simulink model "Remus_AUV_twin"  (R2025b)
settings: Solver=ode4  StartTime=0  StopTime=300  FixedStep=0.1  RelTol=1e-3
undefined symbols (not defined in the file): DiscIntNeverNeededParam
libraries: simulink x1, rllib x1
settings Model: Creator=usdas  LastModifiedBy=OMEN
settings DataIOCC: SaveState=on  InspectSignalLogs=on  ReturnWorkspaceOutputs=off  OutputSaveName=out

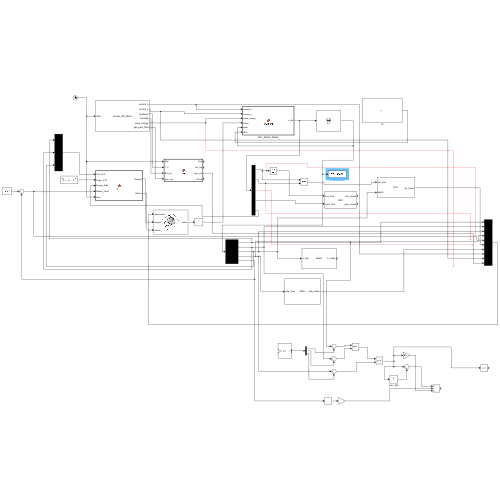
[thumbnail: Simulink's stored preview of the top-level diagram]
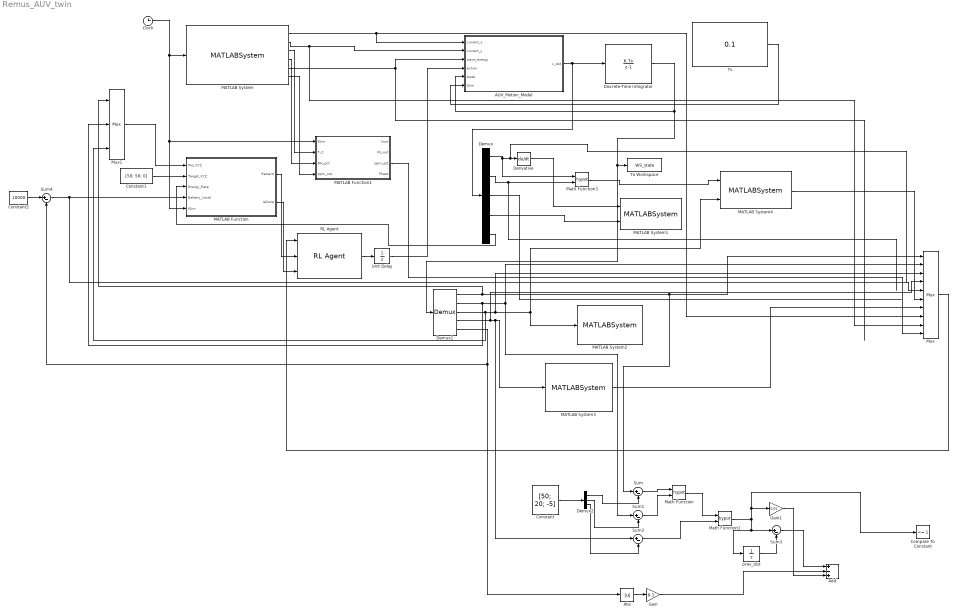
== system Remus_AUV_twin ==
  AUV_Motion_Model : MATLAB Function  TreatAsAtomicUnit=on
  Abs : Abs  SaturateOnIntegerOverflow=off
  Add : Sum  Inputs=+-+
  Clock : Clock
  Compare To Constant : simulink/Logic and Bit Operations/Compare To Constant  relop=<=  const=1  OutDataTypeStr=boolean
  Constant : Constant  Value=[50; 20; -5]  OutDataTypeStr=double  SampleTime=-1
  Constant1 : Constant  Value=[50; 50; 0]
  Constant2 : Constant  Value=10000
  Demux : Demux  Outputs=5
  Demux1 : Demux  Outputs=5
  Demux2 : Demux  Outputs=3
  Derivative : Derivative
  Discrete-Time Integrator : DiscreteIntegrator  InitialCondition=[1;1;0;0;0]  SampleTime=0.1  ICPrevOutput=DiscIntNeverNeededParam  ICPrevScaledInput=DiscIntNeverNeededParam
  Gain : Gain  Gain=0.1
  Gain1 : Gain  Gain=0.01
  MATLAB Function : MATLAB Function  TreatAsAtomicUnit=on
  MATLAB Function1 : MATLAB Function  TreatAsAtomicUnit=on
  MATLAB System : MATLABSystem  System=Ocean_API_Block  SimulateUsing=Interpreted execution
      mask Type: Ocean_API_Block
  MATLAB System1 : MATLABSystem  System=IMU_Block  Ts=0.1  accel_noise=0.02  gyro_noise=0.002  bias_accel=[ 0.05; 0.05; 0.05 ]  bias_gyro=[ 0.002; 0.002; 0.002 ]  SimulateUsing=Code generation
      mask Type: IMU_Block
  MATLAB System2 : MATLABSystem  System=Depth_Block  Ts=0.1  noise=0.02  SimulateUsing=Code generation
      mask Type: Depth_Block
  MATLAB System3 : MATLABSystem  System=Magnetometer_Block  Ts=0.1  yaw_noise=deg2rad( 1.5 )  SimulateUsing=Code generation
      mask Type: Magnetometer_Block
  MATLAB System4 : MATLABSystem  System=DVL_Block  Ts=0.5  noise=0.03  max_depth=60  SimulateUsing=Code generation
      mask Type: DVL_Block
  Math Function : Math  Operator=hypot
  Math Function1 : Math  Operator=hypot
  Math Function3 : Math  Operator=hypot
  Mux : Mux  Inputs=10
  Mux1 : Mux  Inputs=3
  RL Agent : rllib/RL Agent  Agent=agentObj  ExternalActionAsInput=off  ProvideLastAction=off  ProvideCumRwd=off  TreatAsDirectFeedthrough=on  UseStrictObservationDataTypes=off
  Sum{,1..4} (5 alike) : Sum  Inputs=|+-
  To Workspace : ToWorkspace  VariableName=WS_state  SampleTime=0.1
  Ts : Constant  Value=0.1
  Unit Delay : UnitDelay  SampleTime=0.1  HasFrameUpgradeWarning=on
  prev_dist : UnitDelay  InitialCondition=[0, 0, 0]  SampleTime=-1  HasFrameUpgradeWarning=on
  wires:
  Clock/1 -> MATLAB Function1/1(tSim), MATLAB Function/5(tSim), MATLAB System/1
  Discrete-Time Integrator/1 -> Demux1/1, To Workspace/1, AUV_Motion_Model/5(state)
  RL Agent/1 -> Unit Delay/1
  MATLAB System/1 -> Mux/8, AUV_Motion_Model/1(current_x)
  MATLAB System/2 -> Mux/9, AUV_Motion_Model/2(current_y)
  AUV_Motion_Model/1(x_dot) -> Discrete-Time Integrator/1, Demux/1
  Demux/4 -> MATLAB System1/2
  MATLAB System/3 -> MATLAB Function1/2(T_C)
  MATLAB System/4 -> MATLAB Function1/3(RH_pct)
  MATLAB System/6 -> MATLAB Function1/4(ppm_vec)
  MATLAB System/5 -> AUV_Motion_Model/3(wave_energy)
  Ts/1 -> AUV_Motion_Model/6(tSim)
  Demux/1 -> Derivative/1, Math Function3/1
  Derivative/1 -> MATLAB System1/1
  Demux/2 -> Math Function3/2
  Math Function3/1 -> MATLAB System4/1
  Demux1/3 -> Mux1/3, Mux/3, MATLAB System4/2, MATLAB System2/1
  Demux1/4 -> Mux/4, Sum2/1, MATLAB System3/1
  Mux/1 -> RL Agent/1
  Demux1/1 -> Mux1/1, Sum/1, Mux/1
  Demux1/2 -> Mux1/2, Sum1/1, Mux/2
  Demux/3 -> ?
  MATLAB System3/1 -> Mux/7
  Constant/1 -> Demux2/1
  Demux2/1 -> Sum/2
  Demux2/2 -> Sum1/2
  Demux2/3 -> Sum2/2
  Sum/1 -> Math Function/1
  Sum1/1 -> Math Function/2
  Math Function/1 -> Math Function1/1
  Sum2/1 -> Math Function1/2
  Math Function1/1 -> Compare To Constant/1, Gain1/1, prev_dist/1, Sum3/1
  prev_dist/1 -> Sum3/2
  Abs/1 -> Gain/1
  Demux1/5 -> Sum4/2, Abs/1
  Sum3/1 -> Add/1
  Gain/1 -> Add/2
  Gain1/1 -> Add/3
  Mux1/1 -> MATLAB Function/1(Pos_XYZ)
  Constant1/1 -> MATLAB Function/2(Target_XYZ)
  Demux/5 -> MATLAB Function/3(Energy_Rate)
  Constant2/1 -> Sum4/1
  Sum4/1 -> Mux/5, MATLAB Function/4(Battery_Level)
  MATLAB Function/1(Reward) -> RL Agent/2
  MATLAB Function/2(IsDone) -> RL Agent/3
  MATLAB Function1/3(ppm_est) -> Mux/10
  MATLAB System4/1 -> Mux/6
  Unit Delay/1 -> AUV_Motion_Model/4(action)

== matlab function Remus_AUV_twin/MATLAB Function ==
  data: Pos_XYZ input; Reward output; Target_XYZ input; Energy_Rate input; Battery_Level input; tSim input; IsDone output
function [Reward, IsDone] = rewardFcn(Pos_XYZ, Target_XYZ, Energy_Rate, Battery_Level, tSim)
    
    % --- 1. Inputs ---
    dist_to_target = norm(Pos_XYZ(1:2) - Target_XYZ(1:2));
    depth = Pos_XYZ(3);

    % --- 2. Thresholds ---
    dist_threshold = 5.0; 
    max_depth = 60.0;
    max_time = 200;
    
    % --- 3. Calculate Reward (RE-TUNED V3) ---
    
    % A. Distance Progress (Strongest signal: rewards getting closer)
    persistent old_dist
    if isempty(old_dist), old_dist = dist_to_target; end
    
    % r_progress: High reward for moving towards target
    r_progress = (old_dist - dist_to_target) * 20; % INCREASED PROGRESS REWARD
    old_dist = dist_to_target; 
    
    % B. Small Energy Penalty
    r_energy = -0.05 * abs(Energy_Rate); % Reduced from old V2 penalty 
    
    % Total Step Reward
    Reward = r_progress + r_energy;

    % --- 4. Termination ---
    IsDone = 0;
    
    % SUCCESS: Massive Reward
    if dist_to_target < dist_threshold
        Reward = Reward + 1000; 
        IsDone = 1;
    end
    
    % FAILURE: Battery Level / Crash Penalty (NEW PENALTY VALUE: -500)
    if Battery_Level <= 0 && tSim > 0.5 
        Reward = Reward - 500; 
        IsDone = 1;
    end
    
    if depth > max_depth && tSim > 1.0 
        Reward = Reward - 500; % Reduced from -1000
        IsDone = 1;
    end
    
    % TIMEOUT
    if tSim > max_time
        IsDone = 1;
    end
    
    % --- 5. Safety Clamp (NEW PENALTY VALUE: -500) ---
    if (isnan(Reward) || isinf(Reward)) && tSim > 0.5
        Reward = -500; 
        IsDone = 1;
    end
    
    Reward = double(Reward);
    IsDone = double(IsDone);
end

== matlab function Remus_AUV_twin/AUV_Motion_Model ==
  data: current_x input; current_y input; wave_energy input; x_dot output; action input; state input; tSim input
function x_dot = stepImpl(current_x, current_y, wave_energy, action, state, tSim)
% This code has been corrected:
% 1. Removed 'obj.' because this is a MATLAB Function block.
% 2. Added a hard-coded 'drag' variable.
% 3. Fixed the logic for 'v' to include 'yaw_cmd'.

    % --- 0. Define Model Parameters ---
    drag = 0.2; % You can tune this value later

    % --- 1. Extract states ---
    % x = state(1); % Not used
    % y = state(2); % Not used
    % z = state(3); % Not used
    psi = state(4);
    
    % --- 2. Action: Thruster surge + rudder yaw command ---
    u_cmd = action(1);
    yaw_cmd = action(2);

    % --- 3. Hydrodynamic drag influence + current disturbance ---
    % Original code: u = u_cmd - obj.drag * current_x; [cite: 42]
    u = u_cmd - drag * current_x;
    
    % Original code: v = obj.drag * current_y; 
    % Corrected logic (based on original file [cite: 314]):
    v = yaw_cmd - drag * current_y; 

    % --- 4. Base kinematic motion ---
    dx = u * cos(psi) - v * sin(psi);
    dy = u * sin(psi) + v * cos(psi);

    % --- 5. Wave-induced vertical bobbing + lateral drift ---
    dz = 0.05 * sin(0.4 * wave_energy + 0.2*tSim);
    dy = dy + 0.03 * wave_energy; % [cite: 51]

    % --- 6. Heading dynamics ---
    dpsi = 0.05 * yaw_cmd; % [cite: 53]

    % --- 7. Energy Usage Model ---
    energy_used = abs(u_cmd) + abs(yaw_cmd); % [cite: 55]

    % --- 8. Output derivative & energy (5th state) ---
    x_dot = [dx; dy; dz; dpsi; energy_used]; % [cite: 56]
end

== matlab function Remus_AUV_twin/MATLAB Function1 ==
  data: tSim input; Vout output; T_C input; RH_pct input; ppm_vec input; Rs_out output; ppm_est output; Pheat output
function [Vout, Rs_out, ppm_est, Pheat] = fcn(tSim, T_C, RH_pct, ppm_vec)
    % MQ-2 Gas Sensor Logic (Scalar-Safe Version)

    % --- 1. Define Constants ---
    Vc = 5.0;
    RL = 10e3;
    R0 = 10e3;
    C0 = 1000;
    Ts = 0.1;
    tau_resp = 15.0;
    tau_rec  = 45.0;
    alpha_T = -0.004;
    alpha_H = 0.003;
    sigma_Rs = 0.02;
    HeaterPower_W = 0.75;
    Warmup_s = 60;
    
    % Gas Coefficients
    a_LPG = 1.0; b_LPG = 0.45;
    a_CH4 = 1.4; b_CH4 = 0.40;
    a_H2  = 0.8; b_H2  = 0.42;
    a_CO  = 1.8; b_CO  = 0.36;
    w_LPG = 1.0; w_CH4 = 0.7; w_H2 = 0.6; w_CO = 0.3;

    % --- 2. Handle State Memory ---
    persistent Rs warmed
    if isempty(Rs)
        Rs = R0;       
        warmed = 0;    
    end

    % --- 3. Physics Logic (THE FIX IS HERE) ---
    % Check if input is a single number (Scalar) or a list (Vector)
    if isscalar(ppm_vec)
        % If Scalar: Assume the one input is LPG, set others to near-zero
        C_LPG = max(ppm_vec(1), 1e-6);
        C_CH4 = 1e-6; 
        C_H2  = 1e-6;
        C_CO  = 1e-6;
    else
        % If Vector: Unpack all 4 gases normally
        C_LPG = max(ppm_vec(1), 1e-6);
        C_CH4 = max(ppm_vec(2), 1e-6);
        C_H2  = max(ppm_vec(3), 1e-6);
        C_CO  = max(ppm_vec(4), 1e-6);
    end

    % Calculate Target Resistance
    RsL = R0 * a_LPG * C_LPG^(-b_LPG);
    RsM = R0 * a_CH4 * C_CH4^(-b_CH4);
    RsH = R0 * a_H2  * C_H2^(-b_H2);
    RsC = R0 * a_CO  * C_CO^(-b_CO);

    Gmix = w_LPG/RsL + w_CH4/RsM + w_H2/RsH + w_CO/RsC;
    Rs_mix = 1 / max(Gmix, 1e-9);

    % Temp/Humidity Correction
    fT  = 1 + alpha_T * (T_C - 25);
    fRH = 1 + alpha_H * (RH_pct - 65);
    Rs_corr = Rs_mix * fT * fRH;

    % Warmup Logic
    if warmed == 0 && tSim >= Warmup_s
        warmed = 1;
    end
    
    if warmed == 0
        Rs_target = max(Rs_corr, R0 * 10);
    else
        Rs_target = Rs_corr;
    end

    % Dynamics
    if Rs_target < Rs
        tau = tau_resp;
    else
        tau = tau_rec;
    end
    alpha = exp(-Ts / max(tau, 1e-3));
    Rs_next = alpha * Rs + (1 - alpha) * Rs_target;

    % Output Calculation
    Rs_noisy = max(200, Rs_next * (1 + sigma_Rs * randn()));
    Vout = Vc * (RL / (RL + Rs_noisy));
    Rs_out = Rs_noisy;
    ppm_est = C0 * ((Rs_out / R0) / a_LPG)^(-1 / b_LPG);
    Pheat = HeaterPower_W;

    % Update State
    Rs = Rs_next;
end
